simulink model "preshaping2"  (R2024b)
settings: Solver=VariableStepAuto  StartTime=0.0  StopTime=2  RelTol=1e-3
values from neighbouring files (symbols this model uses):
  tau = 0.1    [simulate_preshaping.m]
  wn = 100    [simulate_preshaping.m]
  zeta = 0.05    [simulate_preshaping.m]
settings Model: Creator=shohei  LastModifiedBy=shohei

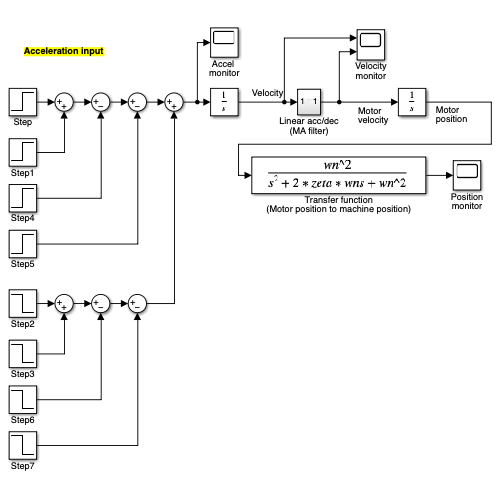
[thumbnail: Simulink's stored preview of the top-level diagram]
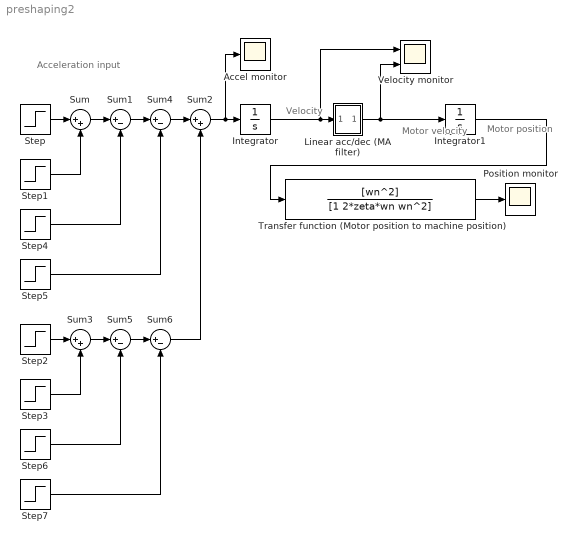
== system preshaping2 ==
  note: Motor
      | velocity
  note: Motor
      | position
  note: Velocity
  note: Acceleration input
  Accel monitor : Scope
  Integrator : Integrator
  Integrator1 : Integrator
  Linear acc/dec (MA filter) : Subsystem
  Position monitor : Scope
  Step : Step  Time=0.1  After=9  SampleTime=0
  Step1 : Step  Time=0.1315  After=6  SampleTime=0
  Step2 : Step  Time=1.1  After=-9  SampleTime=0
  Step3 : Step  Time=1.1315  After=-6  SampleTime=0
  Step4 : Step  Time=0.1628  After=8  SampleTime=0
  Step5 : Step  Time=0.1943  After=7  SampleTime=0
  Step6 : Step  Time=1.1628  After=-8  SampleTime=0
  Step7 : Step  Time=1.1943  After=-7  SampleTime=0
  Sum : Sum  Inputs=|++
  Sum{1,4..6} (4 alike) : Sum  Inputs=|+-
  Sum2 : Sum  Inputs=|++
  Sum3 : Sum  Inputs=|++
  Transfer function (Motor position to machine position) : TransferFcn  Numerator=[wn^2]  Denominator=[1 2*zeta*wn wn^2]
  Velocity monitor : Scope  NumInputPorts=2
  wires:
  Integrator1/1 -> Transfer function (Motor position to machine position)/1
  Linear acc/dec (MA filter)/1(Out1) -> Integrator1/1, Velocity monitor/2
  Sum2/1 -> Accel monitor/1, Integrator/1
  Integrator/1 -> Velocity monitor/1, Linear acc/dec (MA filter)/1(In1)
  Transfer function (Motor position to machine position)/1 -> Position monitor/1
  Step1/1 -> Sum/2
  Step/1 -> Sum/1
  Sum/1 -> Sum1/1
  Step4/1 -> Sum1/2
  Sum1/1 -> Sum4/1
  Sum4/1 -> Sum2/1
  Step5/1 -> Sum4/2
  Sum5/1 -> Sum6/1
  Step2/1 -> Sum3/1
  Sum3/1 -> Sum5/1
  Step3/1 -> Sum3/2
  Step7/1 -> Sum6/2
  Step6/1 -> Sum5/2
  Sum6/1 -> Sum2/2

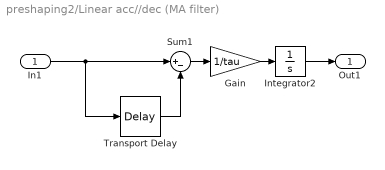
== system preshaping2/Linear acc//dec (MA filter) ==
  In1 : Inport
  Gain : Gain  Gain=1/tau
  Integrator2 : Integrator
  Sum1 : Sum  Inputs=|+-
  Transport Delay : TransportDelay  DelayTime=tau
  Out1 : Outport
  wires:
  In1/1 -> Sum1/1, Transport Delay/1
  Integrator2/1 -> Out1/1
  Gain/1 -> Integrator2/1
  Sum1/1 -> Gain/1
  Transport Delay/1 -> Sum1/2
